simulink library "pathFollowingController_cl"  (R2018b)
settings: Solver=VariableStepAuto  StartTime=0.0  StopTime=10.0  RelTol=1e-3
undefined symbols (not defined in the file or in its folder): env, FLIGHTCONTROLLER, fltCtrl, initializeBussesFromBlock, vhcl
libraries: courseFollow_cl x1, setpointToOutput_cl x1
settings Model: Creator=jldanie5  LastModifiedBy=James Reed

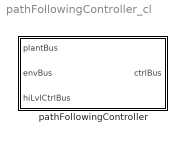
== system pathFollowingController_cl ==
  pathFollowingController : Subsystem  LoadFcn=initializeBussesFromBlock(gcb)  InitFcn=initializeBussesFromBlock(gcb)  StartFcn=initializeBussesFromBlock(gcb)  VariantControl=strcmpi(FLIGHTCONTROLLER,'pathFollowingController')  mask{initPosForInitSStar=vhcl.initPosVecGnd.Value, fluidDensity=env.water.density.Value, pathCtrl=fltCtrl}
      mask prompts: initPosForInitSStar "Initial Position"; fluidDensity "Fluid Density"; pathCtrl "Controller"
      mask init:
      | pathFollowingController_init
      mask DialogControl Container3 Prompt: courseFollow Params
      mask DialogControl Container4 Prompt: setpointToOutput Params

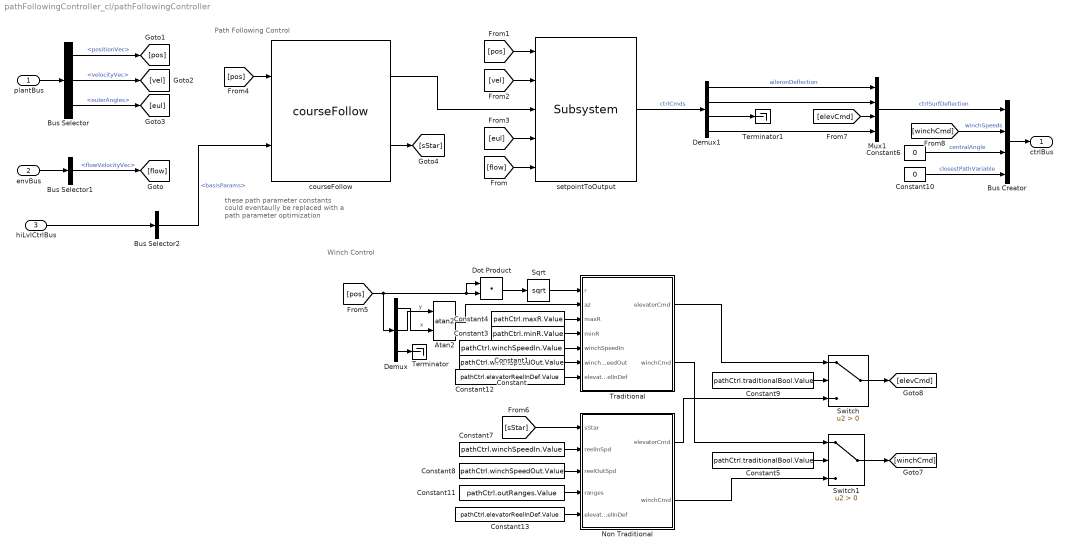
== system pathFollowingController_cl/pathFollowingController ==
  note: Winch Control
  note: these path parameter constants
      | could eventaully be replaced with
      | a path parameter optimization
  note: Path Following Control
  plantBus : Inport  OutDataTypeStr=Bus: plantBus
  envBus : Inport  Port=2  OutDataTypeStr=Bus: envBus
  hiLvlCtrlBus : Inport  Port=3  OutDataTypeStr=Bus: hiLvlCtrlBus
  Atan2 : Trigonometry  Operator=atan2
  Bus Creator : BusCreator  Inputs=4  OutDataTypeStr=Bus: fltCtrlBus
      settings: InheritFromInputs=off
  Bus Selector : BusSelector  OutputSignals=positionVec,velocityVec,eulerAngles
  Bus Selector1 : BusSelector  OutputSignals=flowVelocityVec
  Bus Selector2 : BusSelector  OutputSignals=basisParams
  Constant : Constant  Value=pathCtrl.winchSpeedOut.Value
  Constant1 : Constant  Value=pathCtrl.winchSpeedIn.Value
  Constant10 : Constant  Value=0
  Constant11 : Constant  Value=pathCtrl.outRanges.Value
  Constant12 : Constant  Value=pathCtrl.elevatorReelInDef.Value
  Constant13 : Constant  Value=pathCtrl.elevatorReelInDef.Value
  Constant3 : Constant  Value=pathCtrl.minR.Value
  Constant4 : Constant  Value=pathCtrl.maxR.Value
  Constant5 : Constant  Value=pathCtrl.traditionalBool.Value
  Constant6 : Constant  Value=0
  Constant7 : Constant  Value=pathCtrl.winchSpeedIn.Value
  Constant8 : Constant  Value=pathCtrl.winchSpeedOut.Value
  Constant9 : Constant  Value=pathCtrl.traditionalBool.Value
  Demux : Demux  Outputs=3
  Demux1 : Demux
  Dot Product : DotProduct  InputSameDT=on  OutDataTypeStr=Inherit: Inherit via internal rule
  Mux1 : Mux
  Non Traditional : Stateflow chart  TreatAsAtomicUnit=on
  Sqrt : Sqrt  SaturateOnIntegerOverflow=on
  Switch : Switch  Criteria=u2 > Threshold
  Switch1 : Switch  Criteria=u2 > Threshold
  Terminator : Terminator
  Terminator1 : Terminator
  Traditional : Stateflow chart  TreatAsAtomicUnit=on
  courseFollow : courseFollow_cl/courseFollow  SystemSampleTime=-1
  setpointToOutput : setpointToOutput_cl/Subsystem  SystemSampleTime=-1
  ctrlBus : Outport  OutDataTypeStr=Bus: fltCtrlBus
  wires:
  courseFollow/1 -> setpointToOutput/3
  plantBus/1 -> Bus Selector/1
  Bus Selector/2 -> [vel]  "<velocityVec>"
  Bus Selector/1 -> [pos]  "<positionVec>"
  Bus Selector/3 -> [eul]  "<eulerAngles>"
  [pos] -> setpointToOutput/1
  [vel] -> setpointToOutput/2
  [eul] -> setpointToOutput/4
  [pos] -> courseFollow/1
  Bus Selector2/1 -> courseFollow/2  "<basisParams>"
  Bus Creator/1 -> ctrlBus/1
  envBus/1 -> Bus Selector1/1
  Bus Selector1/1 -> [flow]  "<flowVelocityVec>"
  [flow] -> setpointToOutput/5
  [pos] -> Dot Product/1, Dot Product/2, Demux/1
  Demux/2 -> Atan2/1  "y"
  Demux/1 -> Atan2/2  "x"
  Demux/3 -> Terminator/1
  Dot Product/1 -> Sqrt/1
  Atan2/1 -> Traditional/2(az)
  Mux1/1 -> Bus Creator/1  "ctrlSurfDeflection"
  Constant/1 -> Traditional/6(winchSpeedOut)
  Constant1/1 -> Traditional/5(winchSpeedIn)
  Constant3/1 -> Traditional/4(minR)
  Constant4/1 -> Traditional/3(maxR)
  Sqrt/1 -> Traditional/1(r)
  Demux1/4 -> Mux1/4
  Demux1/2 -> Mux1/2
  Demux1/1 -> Mux1/1  "aileronDeflection"
  setpointToOutput/1 -> Demux1/1  "ctrlCmds"
  [winchCmd] -> Bus Creator/2  "winchSpeeds"
  courseFollow/2 -> [sStar]
  [sStar] -> Non Traditional/1(sStar)
  Constant7/1 -> Non Traditional/2(reelInSpd)
  Constant8/1 -> Non Traditional/3(reelOutSpd)
  Demux1/3 -> Terminator1/1
  Non Traditional/2(winchCmd) -> Switch1/3
  Non Traditional/1(elevatorCmd) -> Switch/3
  [elevCmd] -> Mux1/3
  Traditional/2(winchCmd) -> Switch1/1
  Traditional/1(elevatorCmd) -> Switch/1
  Constant9/1 -> Switch/2
  Constant5/1 -> Switch1/2
  Constant11/1 -> Non Traditional/4(ranges)
  Constant12/1 -> Traditional/7(elevatorReelInDef)
  Constant13/1 -> Non Traditional/5(elevatorReelInDef)
  Switch/1 -> [elevCmd]
  Switch1/1 -> [winchCmd]
  hiLvlCtrlBus/1 -> Bus Selector2/1
  Constant6/1 -> Bus Creator/3  "centralAngle"
  Constant10/1 -> Bus Creator/4  "closestPathVariable"

== stateflow chart pathFollowingController_cl/pathFollowingController/Non Traditional ==
  state ReelIn
    entry:
    elevatorCmd= elevatorReelInDef;
    winchCmd = reelInSpd;
  state ReelOut
    entry:
    winchCmd = reelOutSpd;
    elevatorCmd= 0;
  (default) -> ReelOut
  ReelOut -> ReelIn : [ ~any(and(sStar>=ranges(:,1),sStar<ranges(:,2)))]
  ReelIn -> ReelOut : [any(and(sStar>=ranges(:,1),sStar<ranges(:,2)))]
  data: elevatorCmd output; sStar input; winchCmd output; reelInSpd input; reelOutSpd input; ranges input; elevatorReelInDef input

== stateflow chart pathFollowingController_cl/pathFollowingController/Traditional ==
  state SpoolOut
    entry:
    winchCmd = winchSpeedOut;
    elevatorCmd = 0;
  state SpoolIn
    winchCmd = winchSpeedIn;
    elevatorCmd = elevatorReelInDef;
  (default) -> SpoolIn
  SpoolOut -> SpoolIn : [r > maxR ]
  SpoolIn -> SpoolOut : [r < minR]
  data: elevatorCmd output; r input; az input; winchCmd output; maxR input; minR input; winchSpeedIn input; winchSpeedOut input; elevatorReelInDef input
